simulink model "Nonlinearity"  (R2020b)
settings: Solver=VariableStepAuto  StartTime=0.0  StopTime=tm  RelTol=1e-3
values from neighbouring files (symbols this model uses):
  den = sym2poly(den)    [NonlinearityC.m]    (also in StateSpaceC.m = [1,5,1]; sym2tf.m)
  k = 1    [NonlinearityC.m]
  kp = 0.1    [NonlinearityC.m]    (also in StateSpaceC.m = 1000000)
libraries: simulink x1
settings Model: Creator=huang  LastModifiedBy=huang

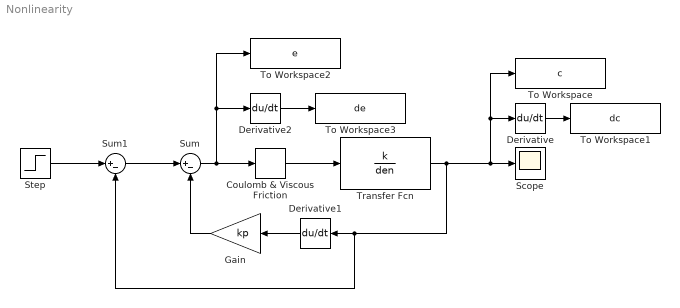
== system Nonlinearity ==
  Coulomb & Viscous Friction : simulink/Discontinuities/Coulomb & Viscous Friction  offset=5.1  gain=0
  Derivative : Derivative
  Derivative1 : Derivative
  Derivative2 : Derivative
  Gain : Gain  Gain=kp
  Scope : Scope
  Step : Step  Time=0  After=0.5  SampleTime=0
  Sum : Sum  Inputs=|+-
  Sum1 : Sum  Inputs=|+-
  To Workspace : ToWorkspace  VariableName=c  SampleTime=-1
      settings: Save2DSignal=2-D array (concatenate along first dimension)
  To Workspace1 : ToWorkspace  VariableName=dc  SampleTime=-1
      settings: Save2DSignal=2-D array (concatenate along first dimension)
  To Workspace2 : ToWorkspace  VariableName=e  SampleTime=-1
      settings: Save2DSignal=2-D array (concatenate along first dimension)
  To Workspace3 : ToWorkspace  VariableName=de  SampleTime=-1
      settings: Save2DSignal=2-D array (concatenate along first dimension)
  Transfer Fcn : TransferFcn  Numerator=k  Denominator=den
  wires:
  Coulomb & Viscous Friction/1 -> Transfer Fcn/1
  Transfer Fcn/1 -> Sum1/2, Derivative1/1, To Workspace/1, Derivative/1, Scope/1
  Derivative/1 -> To Workspace1/1
  Sum1/1 -> Sum/1
  Step/1 -> Sum1/1
  Derivative1/1 -> Gain/1
  Gain/1 -> Sum/2
  Derivative2/1 -> To Workspace3/1
  Sum/1 -> Coulomb & Viscous Friction/1, Derivative2/1, To Workspace2/1
